simulink library "ARBlocks"  (R2017b)
settings: Solver=ode45  StartTime=0.0  StopTime=10.0  RelTol=1e-3  EnableMultiTasking=on
undefined symbols (not defined in the file): sampleTime, ssH, ssPitch, ssPitch2U, ssRoll, ssRoll2V, ssYaw, Standard_Devices, timeDelay, UDP_Protocol, waypoints
libraries: sldrtlib x2, rtwinlib x1
settings Model: Creator=david  LastModifiedBy=ritac
settings DataIOCC: LimitDataPoints=on  SaveFormat=Array
settings OptimizationCC: LifeSpan=inf
settings DebuggingCC: UnderspecifiedInitializationDetection=Classic  MergeDetectMultiDrivingBlocksExec=none  SolverPrmCheckMsg=warning  SFUnexpectedBacktrackingDiag=warning  SFNoUnconditionalDefaultTransitionDiag=warning  SFExecutionAtInitializationDiag=none
settings HardwareCC: ProdBitPerPointer=32  ProdBitPerSizeT=32  ProdBitPerPtrDiffT=32  ProdLargestAtomicFloat=None  ProdIntDivRoundTo=Undefined  ProdEndianess=Unspecified  ProdWordSize=32  ProdHWDeviceType=32-bit Generic
settings ModelReferenceCC: PropagateSignalLabelsOutOfModel=off
settings CodeAppCC: StateflowObjectComments=on
settings GRTTargetCC: TargetLangStandard=C89/C90 (ANSI)  GeneratePreprocessorConditionals=Disable all
settings ConfigComp: CovMetricSettings=dw  CovHtmlReporting=on  CovSaveCumulativeToWorkspaceVar=on  CovSaveSingleToWorkspaceVar=on  CovExternalEMLEnable=off

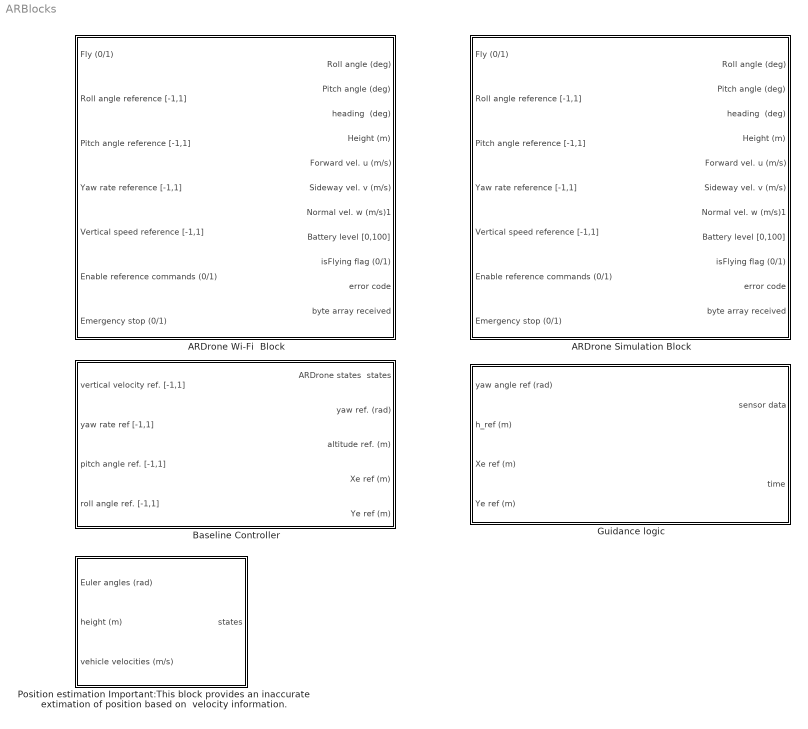
== system ARBlocks ==
  ARDrone Simulation Block : Subsystem
  ARDrone Wi-Fi  Block : Subsystem
  Baseline Controller : Subsystem
  Guidance logic : Subsystem
  "Position estimation Important:This block provides an inaccurate extimation of position based on  velocity information. " : Subsystem

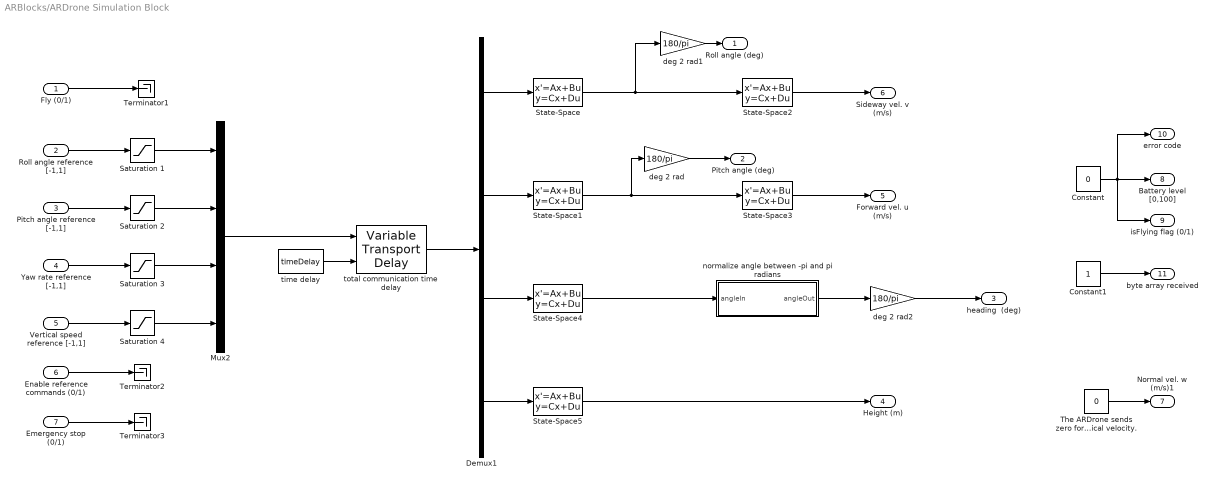
== system ARBlocks/ARDrone Simulation Block ==
  Fly (0/1) : Inport
  Roll angle reference [-1,1] : Inport  Port=2
  Pitch angle reference [-1,1] : Inport  Port=3
  Yaw rate reference [-1,1] : Inport  Port=4
  Vertical speed reference [-1,1] : Inport  Port=5
  Enable reference commands (0/1) : Inport  Port=6
  Emergency stop (0/1) : Inport  Port=7
  Constant : Constant  Value=0
  Constant1 : Constant
  Demux1 : Demux
  Mux2 : Mux
  Saturation {1..4} (4 alike) : Saturate  UpperLimit=1  LowerLimit=-1
  State-Space : StateSpace  A=ssRoll.a  B=ssRoll.b  C=ssRoll.c  D=ssRoll.d  InitialCondition=0
  State-Space1 : StateSpace  A=ssPitch.a  B=ssPitch.b  C=ssPitch.c  D=ssPitch.d  InitialCondition=0
  State-Space2 : StateSpace  A=ssRoll2V.a  B=ssRoll2V.b  C=ssRoll2V.c  D=ssRoll2V.d  InitialCondition=0
  State-Space3 : StateSpace  A=ssPitch2U.a  B=ssPitch2U.b  C=ssPitch2U.c  D=ssPitch2U.d  InitialCondition=0
  State-Space4 : StateSpace  A=ssYaw.a  B=ssYaw.b  C=ssYaw.c  D=ssYaw.d  InitialCondition=0
  State-Space5 : StateSpace  A=ssH.a  B=ssH.b  C=ssH.c  D=ssH.d  InitialCondition=0
  Terminator1 : Terminator
  Terminator2 : Terminator
  Terminator3 : Terminator
  "The ARDrone sends zero for the vertical velocity. " : Constant  Value=0
  deg 2 rad : Gain  Gain=180/pi
  deg 2 rad1 : Gain  Gain=180/pi
  deg 2 rad2 : Gain  Gain=180/pi
  normalize angle between -pi and pi radians : MATLAB Function  TreatAsAtomicUnit=on
  time delay : Constant  Value=timeDelay
  total communication time delay : VariableTransportDelay  MaximumDelay=10  InitialOutput=[0 0 0 0]  MaximumPoints=4096
  Roll angle (deg) : Outport
  Pitch angle (deg) : Outport  Port=2
  heading  (deg) : Outport  Port=3
  Height (m) : Outport  Port=4
  Forward vel. u (m/s) : Outport  Port=5
  Sideway vel. v (m/s) : Outport  Port=6
  Normal vel. w (m/s)1 : Outport  Port=7
  Battery level [0,100] : Outport  Port=8
  isFlying flag (0/1) : Outport  Port=9
  error code : Outport  Port=10
  byte array received : Outport  Port=11
  wires:
  Roll angle reference [-1,1]/1 -> Saturation 1/1
  Pitch angle reference [-1,1]/1 -> Saturation 2/1
  Yaw rate reference [-1,1]/1 -> Saturation 3/1
  Vertical speed reference [-1,1]/1 -> Saturation 4/1
  Demux1/1 -> State-Space/1
  Demux1/4 -> State-Space5/1
  State-Space/1 -> deg 2 rad1/1, State-Space2/1
  State-Space1/1 -> deg 2 rad/1, State-Space3/1
  time delay/1 -> total communication time delay/2
  Mux2/1 -> total communication time delay/1
  total communication time delay/1 -> Demux1/1
  Saturation 1/1 -> Mux2/1
  Saturation 2/1 -> Mux2/2
  Saturation 3/1 -> Mux2/3
  Saturation 4/1 -> Mux2/4
  Demux1/2 -> State-Space1/1
  Demux1/3 -> State-Space4/1
  State-Space4/1 -> normalize angle between -pi and pi radians/1(angleIn)
  Fly (0/1)/1 -> Terminator1/1
  Enable reference commands (0/1)/1 -> Terminator2/1
  Emergency stop (0/1)/1 -> Terminator3/1
  State-Space2/1 -> Sideway vel. v (m/s)/1
  State-Space3/1 -> Forward vel. u (m/s)/1
  State-Space5/1 -> Height (m)/1
  normalize angle between -pi and pi radians/1(angleOut) -> deg 2 rad2/1
  Constant/1 -> isFlying flag (0/1)/1, error code/1, Battery level [0,100]/1
  deg 2 rad/1 -> Pitch angle (deg)/1
  deg 2 rad1/1 -> Roll angle (deg)/1
  deg 2 rad2/1 -> heading  (deg)/1
  Constant1/1 -> byte array received/1
  "The ARDrone sends zero for the vertical velocity. "/1 -> Normal vel. w (m/s)1/1

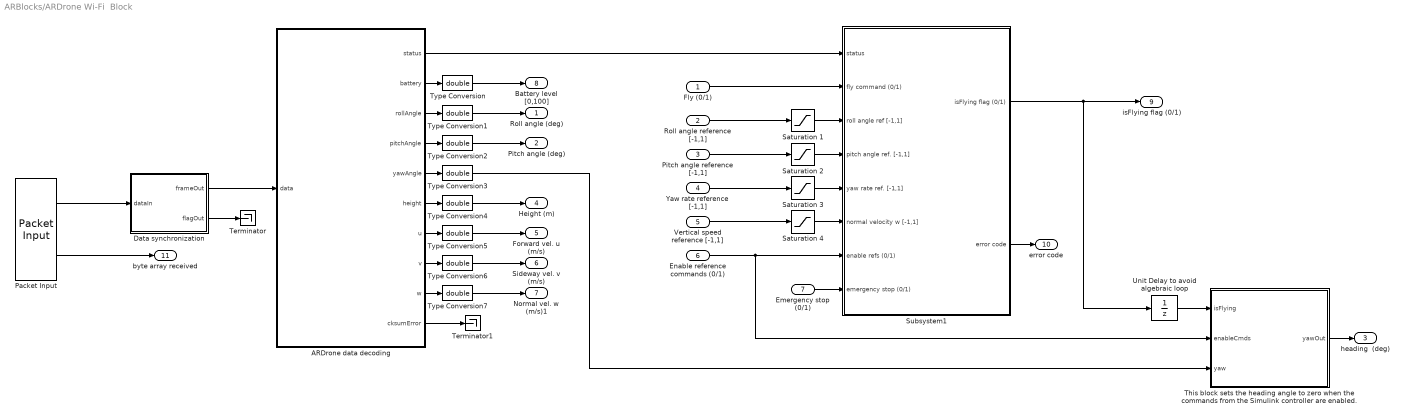
== system ARBlocks/ARDrone Wi-Fi  Block ==
  Fly (0/1) : Inport
  Roll angle reference [-1,1] : Inport  Port=2
  Pitch angle reference [-1,1] : Inport  Port=3
  Yaw rate reference [-1,1] : Inport  Port=4
  Vertical speed reference [-1,1] : Inport  Port=5
  Enable reference commands (0/1) : Inport  Port=6
  Emergency stop (0/1) : Inport  Port=7
  ARDrone data decoding : MATLAB Function  TreatAsAtomicUnit=on
  "Data synchronization " : MATLAB Function  TreatAsAtomicUnit=on
  Packet Input : sldrtlib/Packet Input  SampleTime=sampleTime  MaxMissedTicks=1  ShowMissedTicks=off  YieldWhenWaiting=off  DrvName=Standard_Devices/UDP_Protocol  DrvAddress=5554  DrvOptions=[3232235777 5554]  PacketSize=500  DataTypes='500*uint8'  ShowReady=on  ShowError=off  PacketID=1  ByteOrder=1  ShowTimestamp=off
      settings: AttributesFormatString=Standard Devices\nUDP Protocol [15B2h]  SourceProductName=Simulink Desktop Real-Time
  Saturation {1..4} (4 alike) : Saturate  UpperLimit=1  LowerLimit=-1
  Subsystem1 : Subsystem
  Terminator : Terminator
  Terminator1 : Terminator
  "This block sets the heading angle to zero when the commands from the Simulink controller are enabled. " : MATLAB Function  TreatAsAtomicUnit=on
  Type Conversion{,1..7} (8 alike) : DataTypeConversion  OutDataTypeStr=double
  Unit Delay to avoid algebraic loop : UnitDelay  SampleTime=-1
  Roll angle (deg) : Outport
  Pitch angle (deg) : Outport  Port=2
  heading  (deg) : Outport  Port=3
  Height (m) : Outport  Port=4
  Forward vel. u (m/s) : Outport  Port=5
  Sideway vel. v (m/s) : Outport  Port=6
  Normal vel. w (m/s)1 : Outport  Port=7
  Battery level [0,100] : Outport  Port=8
  isFlying flag (0/1) : Outport  Port=9
  error code : Outport  Port=10
  byte array received : Outport  Port=11
  wires:
  Packet Input/1 -> "Data synchronization "/1(dataIn)
  "Data synchronization "/1(frameOut) -> ARDrone data decoding/1(data)
  ARDrone data decoding/5(yawAngle) -> Type Conversion3/1
  ARDrone data decoding/2(battery) -> Type Conversion/1
  ARDrone data decoding/6(height) -> Type Conversion4/1
  ARDrone data decoding/3(rollAngle) -> Type Conversion1/1
  ARDrone data decoding/4(pitchAngle) -> Type Conversion2/1
  ARDrone data decoding/7(u) -> Type Conversion5/1
  ARDrone data decoding/8(v) -> Type Conversion6/1
  ARDrone data decoding/9(w) -> Type Conversion7/1
  Packet Input/2 -> byte array received/1
  ARDrone data decoding/1(status) -> Subsystem1/1(status)
  Roll angle reference [-1,1]/1 -> Saturation 1/1
  Pitch angle reference [-1,1]/1 -> Saturation 2/1
  Yaw rate reference [-1,1]/1 -> Saturation 3/1
  Vertical speed reference [-1,1]/1 -> Saturation 4/1
  Enable reference commands (0/1)/1 -> "This block sets the heading angle to zero when the commands from the Simulink controller are enabled. "/2(enableCmds), Subsystem1/7(enable refs (0/1))
  Emergency stop (0/1)/1 -> Subsystem1/8(emergency stop (0/1))
  Subsystem1/1(isFlying flag (0/1)) -> isFlying flag (0/1)/1, Unit Delay to avoid algebraic loop/1
  Subsystem1/2(error code) -> error code/1
  ARDrone data decoding/10(cksumError) -> Terminator1/1
  Type Conversion/1 -> Battery level [0,100]/1
  Type Conversion1/1 -> Roll angle (deg)/1
  Type Conversion2/1 -> Pitch angle (deg)/1
  Type Conversion4/1 -> Height (m)/1
  Type Conversion5/1 -> Forward vel. u (m/s)/1
  Type Conversion6/1 -> Sideway vel. v (m/s)/1
  Type Conversion7/1 -> Normal vel. w (m/s)1/1
  Type Conversion3/1 -> "This block sets the heading angle to zero when the commands from the Simulink controller are enabled. "/3(yaw)
  "This block sets the heading angle to zero when the commands from the Simulink controller are enabled. "/1(yawOut) -> heading  (deg)/1
  Fly (0/1)/1 -> Subsystem1/2(fly command (0/1))
  Saturation 1/1 -> Subsystem1/3(roll angle ref [-1,1])
  Saturation 2/1 -> Subsystem1/4(pitch angle ref. [-1,1])
  Saturation 3/1 -> Subsystem1/5(yaw rate ref. [-1,1])
  Saturation 4/1 -> Subsystem1/6(normal velocity w [-1,1])
  "Data synchronization "/2(flagOut) -> Terminator/1
  Unit Delay to avoid algebraic loop/1 -> "This block sets the heading angle to zero when the commands from the Simulink controller are enabled. "/1(isFlying)

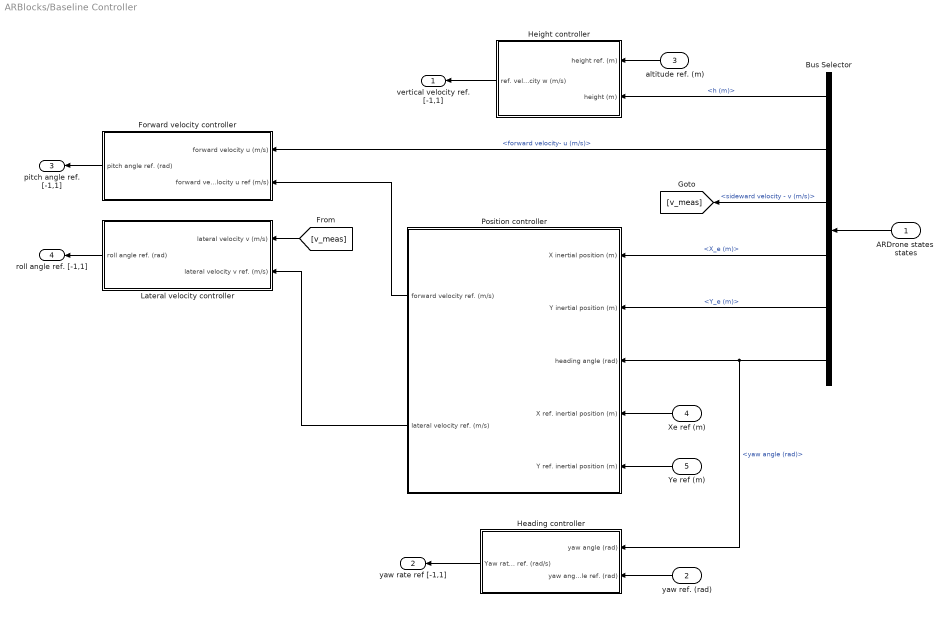
== system ARBlocks/Baseline Controller ==
  "ARDrone states  states " : Inport
  yaw ref. (rad) : Inport  Port=2
  altitude ref. (m) : Inport  Port=3
  Xe ref (m) : Inport  Port=4
  Ye ref (m) : Inport  Port=5
  Bus Selector : BusSelector  OutputSignals=h (m),forward velocity- u (m/s),sideward velocity - v (m/s),X_e (m),Y_e (m),yaw angle (rad)
  "Forward velocity controller " : Subsystem
  Heading controller : Subsystem
  "Height controller " : Subsystem
  Lateral velocity controller : Subsystem
  Position controller : Subsystem
  vertical velocity ref. [-1,1] : Outport
  yaw rate ref [-1,1] : Outport  Port=2
  pitch angle ref. [-1,1] : Outport  Port=3
  roll angle ref. [-1,1] : Outport  Port=4
  wires:
  Bus Selector/6 -> Heading controller/1(yaw angle (rad)), Position controller/3(heading angle (rad))  "<yaw angle (rad)>"
  "ARDrone states  states "/1 -> Bus Selector/1
  altitude ref. (m)/1 -> "Height controller "/1(height ref. (m))
  Bus Selector/1 -> "Height controller "/2(height (m))  "<h (m)>"
  "Height controller "/1(ref. velocity w (m/s)) -> vertical velocity ref. [-1,1]/1
  Lateral velocity controller/1(roll angle ref. (rad)) -> roll angle ref. [-1,1]/1
  Bus Selector/2 -> "Forward velocity controller "/1(forward velocity u (m/s))  "<forward velocity- u (m/s)>"
  "Forward velocity controller "/1(pitch angle ref. (rad)) -> pitch angle ref. [-1,1]/1
  yaw ref. (rad)/1 -> Heading controller/2(yaw angle ref. (rad))
  Heading controller/1(Yaw rate ref. (rad/s)) -> yaw rate ref [-1,1]/1
  Bus Selector/4 -> Position controller/1(X inertial position (m))  "<X_e (m)>"
  Bus Selector/5 -> Position controller/2(Y inertial position (m))  "<Y_e (m)>"
  Xe ref (m)/1 -> Position controller/4(X ref. inertial position (m))
  Ye ref (m)/1 -> Position controller/5(Y ref. inertial position (m))
  Position controller/1(forward velocity ref. (m/s)) -> "Forward velocity controller "/2(forward velocity u ref (m/s))
  Position controller/2(lateral velocity ref. (m/s)) -> Lateral velocity controller/2(lateral velocity v ref. (m/s))
  Bus Selector/3 -> [v_meas]  "<sideward velocity - v (m/s)>"
  [v_meas] -> Lateral velocity controller/1(lateral velocity v (m/s))

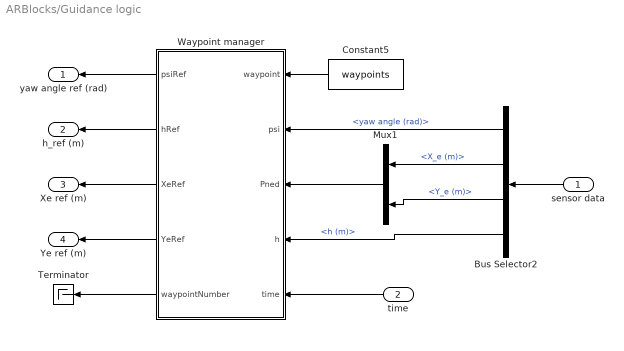
== system ARBlocks/Guidance logic ==
  sensor data : Inport
  time : Inport  Port=2
  Bus Selector2 : BusSelector  OutputSignals=yaw angle (rad),X_e (m),Y_e (m),h (m)
  Constant5 : Constant  Value=waypoints  VectorParams1D=off
  Mux1 : Mux  Inputs=2
  Terminator : Terminator
  "Waypoint manager " : MATLAB Function  TreatAsAtomicUnit=on
  yaw angle ref (rad) : Outport
  h_ref (m) : Outport  Port=2
  Xe ref (m) : Outport  Port=3
  Ye ref (m) : Outport  Port=4
  wires:
  Bus Selector2/2 -> Mux1/1  "<X_e (m)>"
  Bus Selector2/3 -> Mux1/2  "<Y_e (m)>"
  sensor data/1 -> Bus Selector2/1
  Bus Selector2/1 -> "Waypoint manager "/2(psi)  "<yaw angle (rad)>"
  Mux1/1 -> "Waypoint manager "/3(Pned)
  "Waypoint manager "/2(hRef) -> h_ref (m)/1
  "Waypoint manager "/3(XeRef) -> Xe ref (m)/1
  "Waypoint manager "/4(YeRef) -> Ye ref (m)/1
  Bus Selector2/4 -> "Waypoint manager "/4(h)  "<h (m)>"
  time/1 -> "Waypoint manager "/5(time)
  "Waypoint manager "/5(waypointNumber) -> Terminator/1
  "Waypoint manager "/1(psiRef) -> yaw angle ref (rad)/1
  Constant5/1 -> "Waypoint manager "/1(waypoint)

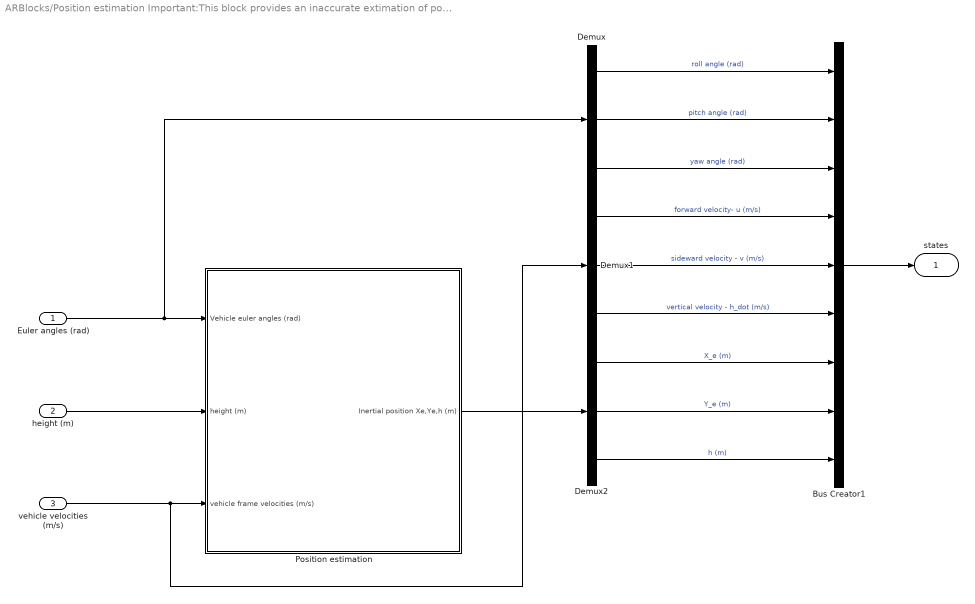
== system ARBlocks/Position estimation Important:This block provides an inaccurate extimation of position based on  velocity information.  ==
  Euler angles (rad) : Inport
  height (m) : Inport  Port=2
  vehicle velocities (m/s) : Inport  Port=3
  Bus Creator1 : BusCreator  Inputs=9
  Demux : Demux  Outputs=3
  Demux1 : Demux  Outputs=3
  Demux2 : Demux  Outputs=3
  Position estimation : Subsystem
  states : Outport
  wires:
  vehicle velocities (m/s)/1 -> Demux1/1, Position estimation/3(vehicle frame velocities (m/s))
  Euler angles (rad)/1 -> Position estimation/1(Vehicle euler angles (rad)), Demux/1
  Position estimation/1(Inertial position Xe,Ye,h (m)) -> Demux2/1
  Demux/1 -> Bus Creator1/1  "roll angle (rad)"
  Demux/2 -> Bus Creator1/2  "pitch angle (rad)"
  Demux/3 -> Bus Creator1/3  "yaw angle (rad)"
  Demux1/1 -> Bus Creator1/4  "forward velocity- u (m/s)"
  Demux1/2 -> Bus Creator1/5  "sideward velocity - v (m/s)"
  Demux1/3 -> Bus Creator1/6  "vertical velocity - h_dot (m/s)"
  Demux2/1 -> Bus Creator1/7  "X_e (m)"
  Demux2/2 -> Bus Creator1/8  "Y_e (m)"
  Demux2/3 -> Bus Creator1/9  "h (m)"
  Bus Creator1/1 -> states/1
  height (m)/1 -> Position estimation/2(height (m))

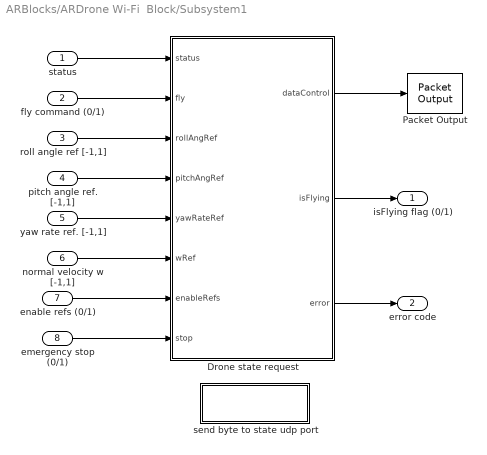
== system ARBlocks/ARDrone Wi-Fi  Block/Subsystem1 ==
  status : Inport
  fly command (0/1) : Inport  Port=2
  roll angle ref [-1,1] : Inport  Port=3
  pitch angle ref. [-1,1] : Inport  Port=4
  yaw rate ref. [-1,1] : Inport  Port=5
  normal velocity w [-1,1] : Inport  Port=6
  enable refs (0/1) : Inport  Port=7
  emergency stop (0/1) : Inport  Port=8
  Drone state request : MATLAB Function  TreatAsAtomicUnit=on  SystemSampleTime=sampleTime
  Packet Output : sldrtlib/Packet Output  SampleTime=-1  MaxMissedTicks=10  ShowMissedTicks=off  YieldWhenWaiting=off  DrvName=Standard_Devices/UDP_Protocol  DrvAddress=5556  DrvOptions=[3232235777 5556]  PacketSize=150  DataTypes='150*uint8'  ShowReady=off  ShowError=off  PacketID=1  ByteOrder=1  InitialValue=[]  FinalValue=[]
      settings: AttributesFormatString=Standard Devices\nUDP Protocol [15B4h]  SourceProductName=Simulink Desktop Real-Time
  "send byte to state udp port " : Subsystem
  isFlying flag (0/1) : Outport
  error code : Outport  Port=2
  wires:
  fly command (0/1)/1 -> Drone state request/2(fly)
  pitch angle ref. [-1,1]/1 -> Drone state request/4(pitchAngRef)
  status/1 -> Drone state request/1(status)
  Drone state request/1(dataControl) -> Packet Output/1
  Drone state request/2(isFlying) -> isFlying flag (0/1)/1
  roll angle ref [-1,1]/1 -> Drone state request/3(rollAngRef)
  yaw rate ref. [-1,1]/1 -> Drone state request/5(yawRateRef)
  normal velocity w [-1,1]/1 -> Drone state request/6(wRef)
  enable refs (0/1)/1 -> Drone state request/7(enableRefs)
  emergency stop (0/1)/1 -> Drone state request/8(stop)
  Drone state request/3(error) -> error code/1

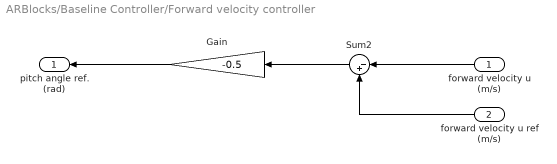
== system ARBlocks/Baseline Controller/Forward velocity controller  ==
  forward velocity u (m/s) : Inport
  forward velocity u ref (m/s) : Inport  Port=2
  Gain : Gain  Gain=-0.5
  Sum2 : Sum  Inputs=|-+
  pitch angle ref. (rad) : Outport
  wires:
  forward velocity u (m/s)/1 -> Sum2/1
  Sum2/1 -> Gain/1
  Gain/1 -> pitch angle ref. (rad)/1
  forward velocity u ref (m/s)/1 -> Sum2/2

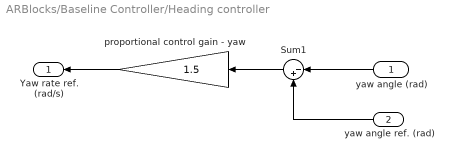
== system ARBlocks/Baseline Controller/Heading controller ==
  yaw angle (rad) : Inport
  yaw angle ref. (rad) : Inport  Port=2
  Sum1 : Sum  Inputs=|-+
  proportional control gain - yaw : Gain  Gain=1.5
  Yaw rate ref. (rad/s) : Outport
  wires:
  yaw angle (rad)/1 -> Sum1/1
  proportional control gain - yaw/1 -> Yaw rate ref. (rad/s)/1
  Sum1/1 -> proportional control gain - yaw/1
  yaw angle ref. (rad)/1 -> Sum1/2

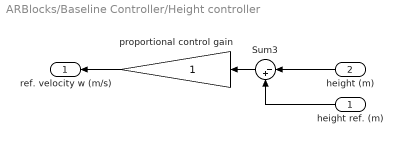
== system ARBlocks/Baseline Controller/Height controller  ==
  height ref. (m) : Inport
  height (m) : Inport  Port=2
  Sum3 : Sum  Inputs=|-+
  proportional control gain : Gain
  ref. velocity w (m/s) : Outport
  wires:
  proportional control gain/1 -> ref. velocity w (m/s)/1
  Sum3/1 -> proportional control gain/1
  height (m)/1 -> Sum3/1
  height ref. (m)/1 -> Sum3/2

== system ARBlocks/Baseline Controller/Lateral velocity controller ==
  lateral velocity v (m/s) : Inport
  lateral velocity v ref. (m/s) : Inport  Port=2
  Gain1 : Gain  Gain=0.4
  Sum5 : Sum  Inputs=|-+
  roll angle ref. (rad) : Outport
  wires:
  lateral velocity v (m/s)/1 -> Sum5/1
  Sum5/1 -> Gain1/1
  Gain1/1 -> roll angle ref. (rad)/1
  lateral velocity v ref. (m/s)/1 -> Sum5/2

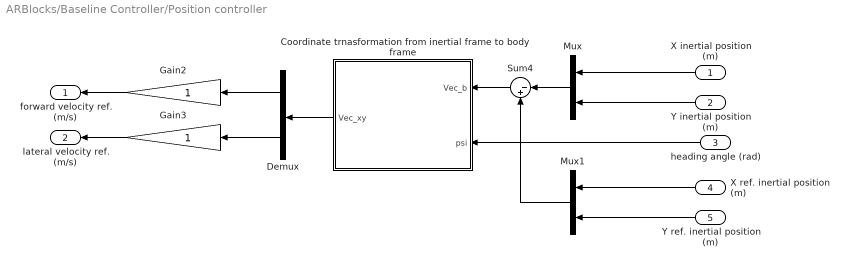
== system ARBlocks/Baseline Controller/Position controller ==
  X inertial position (m) : Inport
  Y inertial position (m) : Inport  Port=2
  heading angle (rad) : Inport  Port=3
  X ref. inertial position (m) : Inport  Port=4
  Y ref. inertial position (m) : Inport  Port=5
  "Coordinate trnasformation from inertial frame to body frame " : MATLAB Function  TreatAsAtomicUnit=on
  Demux : Demux  Outputs=2
  Gain2 : Gain
  Gain3 : Gain
  Mux : Mux  Inputs=2
  Mux1 : Mux  Inputs=2
  Sum4 : Sum  Inputs=|-+
  forward velocity ref. (m/s) : Outport
  lateral velocity ref. (m/s) : Outport  Port=2
  wires:
  Gain2/1 -> forward velocity ref. (m/s)/1
  heading angle (rad)/1 -> "Coordinate trnasformation from inertial frame to body frame "/2(psi)
  "Coordinate trnasformation from inertial frame to body frame "/1(Vec_xy) -> Demux/1
  Mux1/1 -> Sum4/2
  Sum4/1 -> "Coordinate trnasformation from inertial frame to body frame "/1(Vec_b)
  Y inertial position (m)/1 -> Mux/2
  X inertial position (m)/1 -> Mux/1
  Mux/1 -> Sum4/1
  X ref. inertial position (m)/1 -> Mux1/1
  Y ref. inertial position (m)/1 -> Mux1/2
  Demux/1 -> Gain2/1
  Demux/2 -> Gain3/1
  Gain3/1 -> lateral velocity ref. (m/s)/1

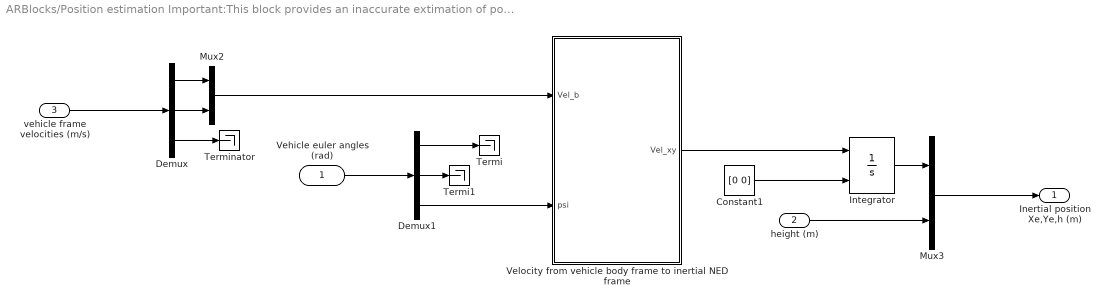
== system ARBlocks/Position estimation Important:This block provides an inaccurate extimation of position based on  velocity information. /Position estimation ==
  Vehicle euler angles (rad) : Inport
  height (m) : Inport  Port=2
  vehicle frame velocities (m/s) : Inport  Port=3
  Constant1 : Constant  Value=[0 0]
  Demux : Demux  Outputs=3
  Demux1 : Demux  Outputs=3
  Integrator : Integrator  InitialConditionSource=external
  Mux2 : Mux  Inputs=2
  Mux3 : Mux  Inputs=2
  Termi : Terminator
  Termi1 : Terminator
  Terminator : Terminator
  Velocity from vehicle body frame to inertial NED  frame : MATLAB Function  TreatAsAtomicUnit=on
  Inertial position Xe,Ye,h (m) : Outport
  wires:
  Demux/3 -> Terminator/1
  Demux/2 -> Mux2/2
  Demux/1 -> Mux2/1
  Mux2/1 -> Velocity from vehicle body frame to inertial NED  frame/1(Vel_b)
  Demux1/1 -> Termi/1
  Demux1/2 -> Termi1/1
  Velocity from vehicle body frame to inertial NED  frame/1(Vel_xy) -> Integrator/1
  Constant1/1 -> Integrator/2
  Integrator/1 -> Mux3/1
  Demux1/3 -> Velocity from vehicle body frame to inertial NED  frame/2(psi)
  vehicle frame velocities (m/s)/1 -> Demux/1
  Vehicle euler angles (rad)/1 -> Demux1/1
  height (m)/1 -> Mux3/2
  Mux3/1 -> Inertial position Xe,Ye,h (m)/1

== system ARBlocks/ARDrone Wi-Fi  Block/Subsystem1/send byte to state udp port  ==
  Constant : Constant  Value=[1 ;13]  OutDataTypeStr=uint8
  Packet Output1 : rtwinlib/Packet Output  SampleTime=sampleTime*10  MaxMissedTicks=10  ShowMissedTicks=off  YieldWhenWaiting=off  DrvName=Standard_Devices/UDP_Protocol  DrvAddress=5554  DrvOptions=[3232235777 5554]  PacketSize=2  DataTypes='2*uint8'  ShowReady=off  ShowError=off  PacketID=1  ByteOrder=1  InitialValue=[]  FinalValue=[]
      settings: AttributesFormatString=Standard Devices\nUDP Protocol [15B2h]  SourceProductName=Simulink Desktop Real-Time  SourceProductBaseCode=WT
  Rate Transition : RateTransition  OutPortSampleTime=sampleTime*10
  wires:
  Constant/1 -> Rate Transition/1
  Rate Transition/1 -> Packet Output1/1

== matlab function ARBlocks/ARDrone Wi-Fi  Block/Subsystem1/Drone state request ==
  data: status input; fly input; rollAngRef input; pitchAngRef input; yawRateRef input; wRef input; enableRefs input; dataControl output; isFlying output; stop input; error output
function [dataControl, isFlying, error] = fcn( status, fly, rollAngRef, pitchAngRef, yawRateRef, wRef, enableRefs, stop)
%#codegen

% Persistent variables.
persistent SequenceNumber ;

% Initialization of persistent variables at first time step. 

if isempty(SequenceNumber)
    SequenceNumber = 1 ;
end



% Error code / No error: 0
error=0;

% Boolean of flying status / Flying: 1
isFlying = status(32) ;

% Byte array of size 150 to be sent to the drone.
strOut = uint8(zeros(150,1)) ;

% String that coontains a variable size command. 
% cmd is concatenated with previous commands at each sample
cmd = '';

% At first time step and every 100 time steps, data is requested.
if (SequenceNumber <=1 || mod(SequenceNumber, 100) ==0 )
    SequenceNumber = SequenceNumber+1; 
    strCmd = getString(SequenceNumber) ;
    cmd = ['AT*CONFIG=' strCmd ',"general:navdata_demo","TRUE"' char(13)];
    
end

SequenceNumber = SequenceNumber+1;
strCmd = getString(SequenceNumber) ;
cmd = [cmd 'AT*COMWDG=' strCmd char(13)];


if stop ==1 % Emergency stop
   cmd = ['AT*REF=' strCmd ',290717952' char(13)] ; 
    
else % Not emergency stop
    
    if SequenceNumber >20 && SequenceNumber <22
        
        % Trim vehicle state estimation / angles set to zero
        SequenceNumber =SequenceNumber+1;
        strCmd = getString(SequenceNumber) ;
        cmd = [cmd 'AT*FTRIM=' strCmd char(13)] ;
        
    elseif SequenceNumber >=22 && SequenceNumber <25
        cmd = [cmd 'AT*CONFIG=' strCmd '"conrol:altitude_max","100000"' char(13)] ;
        
        
    elseif SequenceNumber >=25
        
        if ( fly == 1  )
            
            if (isFlying ==0)
                
                SequenceNumber =SequenceNumber+1;
                strCmd = getString(SequenceNumber) ;
                cmd = [cmd 'AT*REF=' strCmd ',290718208' char(13)] ;
            
            elseif isFlying==1 && enableRefs==1
                
                SequenceNumber =SequenceNumber+1;
                strCmd = getString(SequenceNumber) ;
                      
                cmd = [cmd 'AT*PCMD=' strCmd ',1,'] ;
                 
                aux = double (float2IEEE754 (rollAngRef) )  ;
                strAux = getString(abs(aux)) ; 
                if rollAngRef<0
                   strAux = [char(45) strAux] ; 
                end
                cmd = [cmd strAux ','];
                      
               aux = double (float2IEEE754 (pitchAngRef) ) ;
               strAux = getString(abs(aux)) ; 
               if pitchAngRef<0
                    strAux = [char(45) strAux] ; 
               end
               cmd = [cmd strAux ','];
                      
               aux =  double(float2IEEE754 (wRef)) ;
               strAux = getString(abs(aux)) ; 
               if wRef<0
                    strAux = [char(45) strAux] ; 
               end
               cmd = [cmd strAux ','];
                      
                      
               aux =  double (float2IEEE754 (yawRateRef) ) ;
               strAux = getString(abs(aux)) ; 
               if yawRateRef <0
                     error=2; 
                     strAux = [char(45) strAux] ; 
               end
               cmd = [cmd strAux char(13)];
               
                
            end
            
            
        elseif ( fly==0 )
                
               if isFlying ==1
                    SequenceNumber =SequenceNumber+1;
                    strCmd = getString(SequenceNumber) ;
                    cmd = [cmd 'AT*REF=' strCmd ',290717696' char(13)] ;
                    
               end
        end
        
    end
    
    
    
end

% cmd must contain less than 150 bytes. 
if (length(cmd)<150)
    strOut(1:length(cmd)) = cmd ;
else
    error =1; 
end

dataControl = strOut;

end


%% My str2num function that allows for code generation
function [ strOut] = getString( a )
d=1;

if (a<10)
    d=1;
end

if (a >=10 && a <100)
    d=2;
end

if (a >=100 && a <1000)
    d=3;
end

if (a >=1000 && a <10000)
    d=4;
end

if (a >=10000 && a <100000)
    d=5;
end

if (a >=100000 && a <1000000)
    d=6;
end

if (a >=1000000 && a <10000000)
    d=7;
end

if (a >=10000000 && a <100000000)
    d=8;
end

if (a >=100000000 && a <1000000000)
    d=9;
end

if (a >=1000000000 && a <10000000000)
    d=10;
end

if (a >=10000000000 )
    d=11;
end



digit = uint8(zeros(1,d)) ;
resTotal = 0;
%d = length(a) ;
for k=1:d
    
    res1 = mod(a,10^k)/(10^(k-1)) ;
    %( mod(a,10*k) - resTotal)/(10*k) ;
    
    digit(d-k+1) = char(48 + res1);
    resTotal = (10^(k-1))*res1 +resTotal;
    
end

strOut = char(digit) ;


end

%% Function to obtain a IEEE754 representation of a float number
function [ iVal ] = float2IEEE754( fVal )

binData = dec2bin(typecast (single(fVal), 'uint8'),8) 

binData2 =[ binData(4,:) binData(3,:) binData(2,:) binData(1,:)] 
iVal =0; 
for k=32:-1:1
    
    if (binData2(k) =='1')
        bit = 1;
    else
        bit =0;
    end
    
    if k == 1
        iVal = iVal - bit*2^(31);
    else
        iVal = iVal + bit*2^(32-k) ; 
    end
    
end

iVal = int32(iVal)

end

== matlab function ARBlocks/ARDrone Wi-Fi  Block/ARDrone data decoding ==
  data: status output; battery output; rollAngle output; pitchAngle output; data input; yawAngle output; height output; u output; v output; w output; cksumError output
function [ status, battery,  rollAngle, pitchAngle, yawAngle, height, u,v,w , cksumError ]= fcn(data)
%#codegen

% Checksum array. cksum(1) contains the computed checksum, cksum(2)
% contains the checksum sent by the ARDrone. 
cksum = [0 0 ]; 

% Previous value of height 
persistent hPrev ; 
% Previous data packet
persistent dataPrev ; 

% Initialization of persistent variables
if isempty(hPrev)
    hPrev=0 ; 
end

if isempty(dataPrev)
    dataPrev = uint8(zeros(496,1)) ;
end

% Computing checksum
cksum(1) =  sum(double(data(1:end-8))) +442; 
% Checksum given by the drone
cksum(2) = double(data(end-3)) + double(data(end-2))*256 +  double(data(end-1))*256^2 + double(data(end))*256^3 ; 
% Checksum error
cksumError = abs(cksum(1)-cksum(2));
%% Change the following if statement to ensure that the data checksum is valid 
%if (data(15) == 148 && cksumError==0 )
if (data(15) == 148  )
    dataPrev = data; 
else
    data = dataPrev; 
end

% Converting bytes to drone information
status = getDroneState(data(1:4));
battery = decode(data(21:24),1); % unit: deg
pitchAngle = decode(data(25:28),0)/1000; % unit: deg
rollAngle = decode(data(29:32),0)/1000; % unit: deg
yawAngle = decode(data(33:36),0)/1000; % unit: deg
height = decode(data(37:40),1)/1000; % unit: deg
u = decode(data(41:44),0)/1000; % unit: m/s
v = decode(data(45:48),0)/1000; % unit: m/s
w = decode(data(49:52),0)/1000; % unit: m/s



if (status(32) ==1 && height< 0.2   )
    height = hPrev;
elseif status(32)==1 
    hPrev= height; 
end
  
    
end


function res = decode(input, mark)
% if mark = 1; then output a int
% else output the float value which is defined by SDK description.
% the input is an array (1*4) 
% e.g. : NDS(Battery_OS:Battery_OS+data_length-1)
    hex_value = dec2hex(input);
    hex_value = [hex_value(4,:),hex_value(3,:),hex_value(2,:),hex_value(1,:)];
    if mark ==1
        res = hex2dec(hex_value);
    else
        res = typecast(uint32(hex2dec(hex_value)),'single');
    end
end

function bin = getDroneState(input)
    bin = zeros(32,1); 
    hex = dec2hex(input);
    % put the hex_value in the order [31, 30......0]
    hex = [hex(4,:),hex(3,:),hex(2,:),hex(1,:)];
for i=1:length(hex)
    if hex(i)=='F'
        bin((i*4)-3:i*4)=[1 1 1 1];
    elseif hex(i)=='E'
        bin((i*4)-3:i*4)=[1 1 1 0];
    elseif hex(i)=='D'
        bin((i*4)-3:i*4)=[1 1 0 1];
    elseif hex(i)=='C'
        bin((i*4)-3:i*4)=[1 1 0 0];
    elseif hex(i)=='B'
        bin((i*4)-3:i*4)=[1 0 1 1];
    elseif hex(i)=='A'
        bin((i*4)-3:i*4)=[1 0 1 0];
    elseif hex(i)=='9'
        bin((i*4)-3:i*4)=[1 0 0 1];
    elseif hex(i)=='8'
        bin((i*4)-3:i*4)=[1 0 0 0];
    elseif hex(i)=='7'
        bin((i*4)-3:i*4)=[0 1 1 1];
    elseif hex(i)=='6'
        bin((i*4)-3:i*4)=[0 1 1 0];
    elseif hex(i)=='5'
        bin((i*4)-3:i*4)=[0 1 0 1];
    elseif hex(i)=='4'
        bin((i*4)-3:i*4)=[0 1 0 0];
    elseif hex(i)=='3'
        bin((i*4)-3:i*4)=[0 0 1 1];
    elseif hex(i)=='2'
        bin((i*4)-3:i*4)=[0 0 1 0];
    elseif hex(i)=='1'
        bin((i*4)-3:i*4)=[0 0 0 1];
    elseif hex(i)=='0'
        bin((i*4)-3:i*4)=[0 0 0 0];
    end
end

end

== matlab function ARBlocks/ARDrone Wi-Fi  Block/Data synchronization  ==
  data: dataIn input; frameOut output; flagOut output
function [frameOut,flagOut]  = fcn(dataIn)
%#eml
%% Author: David Escobar Sanabria
%  Description: This function synchronizes data coming from the flight computer
%  computer. 
%  frameOut: Organized frame
%  frameIn: sequence of bytes not sync.
persistent frame; 
persistent lastFrame; 
persistent count; 
persistent countHeader; 
persistent countBuffer; 
persistent buffer; 

%% Size of byte array containing the data
sizePayload= 496;

%% Size of the array read each time step
nBytes = 500 ;%size(dataIn,1); 


%%%%%%%%%%%%%%%%%%%%%%%%%%%%%%%%%%%%%%%%%%%%%%%%%%%%%%%
%% Initialization of presistent variables
if isempty(buffer)
    buffer=uint8(zeros(1024,1));
end

if isempty(countBuffer)
    countBuffer=0;
end


if isempty(frame)
    frame=uint8(zeros(sizePayload,1));
end

if isempty(lastFrame)
    lastFrame=uint8(zeros(sizePayload,1));
end


if isempty(count)
    count=0;
end

if isempty(countHeader)
    countHeader=0;
end
%%%%%%%%%%%%%%%%%%%%%%%%%%%%%%%%%%%%%%%%%%%%%%%%%%%%%%%

%% Filling the buffer
buffer(countBuffer+1:countBuffer+nBytes) = dataIn;

bytesToRead = countBuffer+nBytes; 

%%%%%%%%%%%%%%%%%%%%%%%%%%%%%%%%%%%%%%%%%%%%%%%%%%%%%%%
%% Reading buffer

for k=1:bytesToRead    
    if(countHeader==4 && count<sizePayload)
        bytesLeft = sizePayload-count;
        frame(count+1:sizePayload) = buffer(k:k+bytesLeft-1);
        count = sizePayload;
        countBuffer = bytesToRead-bytesLeft ;
        buffer(1:countBuffer) = buffer(k+bytesLeft:bytesToRead);
        break;
        
    end
    
    if(countHeader==3 && buffer(k)==85)
        
        countHeader=4;
 
        if(bytesToRead-k > sizePayload)
            count =sizePayload;  
            frame(1:count) = buffer(k+1:k+sizePayload);  
            countBuffer =bytesToRead-k-sizePayload ; 
            buffer(1:countBuffer) = buffer(k+sizePayload+1:bytesToRead);
        else
            
            count =bytesToRead-k;
            if count > 0          
                frame(1:count) = buffer(k+1:bytesToRead);  
            end
            countBuffer = 0; 
            
        end
        
        break;
    end
    
    if(countHeader==2 && buffer(k)==102)
        countHeader=3;
    end
    
    if(countHeader==1 && buffer(k)==119)
        countHeader=2;
    end
       
    if(countHeader==0 && buffer(k)==136)
        countHeader=1;
    end

end

if count==sizePayload 
     frameOut = frame;
     flagOut = 1; 
     lastFrame = frame;
     frame=uint8(zeros(sizePayload,1));
     count=0;
     countHeader=0;
     
else % In case the buffer does not have an entire payload
    frameOut = lastFrame;
    flagOut = 0; 
end

== matlab function ARBlocks/ARDrone Wi-Fi  Block/This block sets the heading angle to zero when the commands from the Simulink controller are enabled.  ==
  data: isFlying input; enableCmds input; yawOut output; yaw input
% Description: This function zeroes out the heading angle once the commands
% are enabled. 
function yawOut = fcn(isFlying,enableCmds,yaw)
%#codegen

yawOut = yaw; 
persistent yaw0 ; 
persistent mode ; 

if isempty (yaw0)
yaw0 = 0; 
end


if isempty (mode)
mode=0; 
end

if isFlying ==1 && enableCmds==1    
    yawOut = yaw - yaw0; 
    mode =1; 
elseif isFlying ==1 && mode ==0
    yaw0 = yaw; 
end


yawOut = mod(yawOut, 360) ;
if yawOut > 180
    yawOut = -360 + yawOut ; 
end

== matlab function ARBlocks/ARDrone Simulation Block/normalize angle between -pi and pi radians ==
  data: angleIn input; angleOut output
function angleOut = fcn(angleIn)
%#codegen

angleOut = mod(angleIn, 2*pi) ;
if angleOut > pi
    angleOut = -2*pi + angleOut ; 
end

== matlab function ARBlocks/Position estimation Important:This block provides an inaccurate extimation of position based on  velocity information. /Position estimation/Velocity from vehicle body frame to inertial NED  frame ==
  data: Vel_b input; Vel_xy output; psi input
function Vel_xy = fcn(Vel_b , psi)
%#codegen
Vel_xy = zeros(2,1);
T = [cos(psi) -sin(psi) ; sin(psi) cos(psi)] ; 
Vel_xy = T*Vel_b;

== matlab function ARBlocks/Baseline Controller/Position controller/Coordinate trnasformation from inertial frame to body frame  ==
  data: Vec_b input; Vec_xy output; psi input
function Vec_xy  = fcn(Vec_b , psi)
%#codegen
T = [cos(psi) sin(psi) ; -sin(psi) cos(psi)] ; 
Vec_xy = T*Vec_b(1:2,1);

== matlab function ARBlocks/Guidance logic/Waypoint manager  ==
  data: psiRef output; hRef output; waypoint input; psi input; Pned input; h input; XeRef output; YeRef output; time input; waypointNumber output
function [psiRef, hRef,  XeRef, YeRef, waypointNumber]       = fcn(waypoint, psi, Pned, h, time )
%#codegen

% Waypoint matrix contains final position, orientatoin, and waiting time.

% Number of waypoints
nPoints = size(waypoint, 2) ;

% Persitent variable used to keep trak of next waypoint
persistent wpointer;

% Time zero for each waypoint. This is used to wait at a desired position.
persistent t0 ;

% Init. persistent variables
if isempty(wpointer)
    wpointer = 1;
end

if isempty(t0)
    t0 = 0;
end

% A waypoint is reached if the distance between the desired waypoint and 
% the vehicle is less than 0.3 m in the XY plane, less than 0.3 m in height, 
% and less than 5 degrees in  heading. 

if ( norm(Pned(1:2,1) - waypoint(1:2, wpointer) )< 0.3 && ...
        norm(h - waypoint(3, wpointer)) < 0.3  && norm(psi - waypoint(4, wpointer) )< 5*pi/180   )
    
    if(wpointer ~= nPoints)
        
        if (t0 ==0)
            t0 = time;
        else
            if (time - t0 > waypoint(5, wpointer))
                
                 if(wpointer < nPoints)
                    wpointer = wpointer+ 1;
                    t0 = 0;
                 end
                
            end
        end
        
             
    end
    
       
    
end


%% Outputs:
hRef = waypoint(3, wpointer) ;
psiRef = waypoint(4, wpointer) ;
XeRef = waypoint(1, wpointer) ;
YeRef = waypoint(2, wpointer) ;
waypointNumber = wpointer ;
